simulink model "ex_full_state_feedback_model"  (R2024b)
settings: Solver=VariableStepAuto  StartTime=0.0  StopTime=30  RelTol=1e-3
PreLoadFcn:
  | % time constant
  | tc = 1.5;
InitFcn:
  | % initial states
  | X0 = [1;1;1];
  | 
  | % system matrices
  | A = [-0.14 0.33 -0.33; 0.1 -0.28 0; 0 1.7 -0.77];
  | B = [0; 0; -0.025];
  | C = [2 0 0];
  | 
  | % desired eigenvalues
  | epsilon = [0 1e-4 -1e-4];
  | E = [-1/tc -1/tc -1/tc]+epsilon;
  | 
  | % closed-loop pole assignment using state feedback
  | [K,PREC] = place(A,B,E);
StartFcn:
  | % desired eigenvalues
  | epsilon = [0 1e-4 -1e-4];
  | E = [-1/tc -1/tc -1/tc]+epsilon;
  | 
  | % closed-loop pole assignment using state feedback
  | [K,PREC] = place(A,B,E);
values from neighbouring files (symbols this model uses):
  K = place(A,B,E1(1:3))    [ex_integral_control.m]    (also in ex_specifications.m = place(A,B,E); ex_water.m = K1(:,1:n); ex_water_tank.m = K1(:,1:n))
settings Model: Creator=Dan  LastModifiedBy=Dan

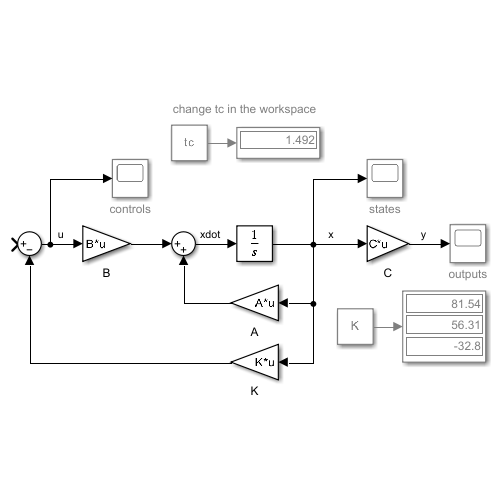
[thumbnail: Simulink's stored preview of the top-level diagram]
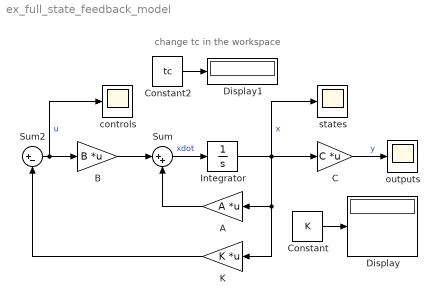
== system ex_full_state_feedback_model ==
  note: change tc in the workspace
  A : Gain  Gain=A  Multiplication=Matrix(K*u)
  B : Gain  Gain=B  Multiplication=Matrix(K*u)
  C : Gain  Gain=C  Multiplication=Matrix(K*u)
  Constant : Constant  Value=K
  Constant2 : Constant  Value=tc
  Display : Display
  Display1 : Display
  Integrator : Integrator  InitialCondition=X0
  K : Gain  Gain=K  Multiplication=Matrix(K*u)
  Sum : Sum  Inputs=|++
  Sum2 : Sum  Inputs=|+-
  controls : Scope
  outputs : Scope
  states : Scope
  wires:
  Sum2/1 -> B/1, controls/1  "u"
  Sum/1 -> Integrator/1  "xdot"
  B/1 -> Sum/1
  Integrator/1 -> states/1, C/1, K/1, A/1  "x"
  A/1 -> Sum/2
  C/1 -> outputs/1  "y"
  K/1 -> Sum2/2
  Constant/1 -> Display/1
  Constant2/1 -> Display1/1
